simulink model "Hamiltonian_model"  (R2018b)
settings: Solver=FixedStepAuto  StartTime=0.0  StopTime=tsim  FixedStep=T  RelTol=1e-3
values from neighbouring files (symbols this model uses):
  a1 = 6.5035    [DoD_simulation.m]    (also in Hamiltonian_sim.m)
  a2 = 6.3853e-4    (= 0.00063853)    [DoD_simulation.m]    (also in Hamiltonian_sim.m)
  a3 = 0.0011    [DoD_simulation.m]    (also in Hamiltonian_sim.m)
  a4 = 0.0250    (= 0.025)    [DoD_simulation.m]    (also in Hamiltonian_sim.m)
  a5 = 0.1042    [DoD_simulation.m]    (also in Hamiltonian_sim.m)
  a6 = 0.0012    [DoD_simulation.m]    (also in Hamiltonian_sim.m)
  Aineq = [eye(N_MPC);-eye(N_MPC)]    [Hamiltonian_sim.m]
  B1 = 3.0021e3    (= 3002.1)    [DoD_simulation.m]    (also in Hamiltonian_sim.m)
  B2 = 986.7121    [DoD_simulation.m]    (also in Hamiltonian_sim.m)
  B3 = 210000    [DoD_simulation.m]    (also in Hamiltonian_sim.m)
  B4 = 19998    [DoD_simulation.m]    (also in Hamiltonian_sim.m)
  B5 = 35000    [DoD_simulation.m]    (also in Hamiltonian_sim.m)
  B6 = 19998    [DoD_simulation.m]    (also in Hamiltonian_sim.m)
  bineq = [fracU_max; -fracU_min]    [Hamiltonian_sim.m]
  Cm = [0, 0, 1, 0 ... (first row only)    [DoD_simulation.m]    (also in Hamiltonian_sim.m = [1, 0, 0, 0)
  Dm = [0;0;0]    [DoD_simulation.m]    (also in Hamiltonian_sim.m = [0; 0; 0])
  g = 9.82    [DoD_simulation.m]    (also in Hamiltonian_sim.m)
  Gamma = WW.'*[(BB.'*QQ + SS.')*(AA + BB*EE) + (BB.'*SS + RR)*EE, -(BB.'*QQ + SS.')*kron(ones(N_MPC+1,1),NN)]    [Hamiltonian_sim.m]
  Jo = 0.5*mo*(ro^2)    (= 0.000244290244743)    [DoD_simulation.m]    (also in Hamiltonian_sim.m)
  k = place(Ac,Bc,[p1 p2 p3])    [Hamiltonian_sim.m]
  Kc = zeros(1,length(idx))    [DoD_simulation.m]    (also in Hamiltonian_sim.m)
  Kw = 0.0086    [DoD_simulation.m]    (also in Hamiltonian_sim.m)
  Linv = L_H\eye(size(H,1))    [Hamiltonian_sim.m]
  Lo = dlqr(Aod.',Cm.',Qo,Ro).'    [DoD_simulation.m]
  mo = pi*(ro^2)*thick*p    (= 0.135716802635)    [DoD_simulation.m]    (also in Hamiltonian_sim.m)
  mup_init = [0; 0; theta0; phi0]    [DoD_simulation.m]    (also in Hamiltonian_sim.m)
  N = 98.78    [DoD_simulation.m]    (also in Hamiltonian_sim.m)
  n_in = size(Bcd,2)    [Hamiltonian_sim.m]
  n_out = size(Cc,1)    [Hamiltonian_sim.m]
  Nu = NN(end)    [DoD_simulation.m]    (also in Hamiltonian_sim.m)
  Nx = zeros(length(Cr),1)    [DoD_simulation.m]    (also in Hamiltonian_sim.m)
  opt = mpcqpsolverOptions    [Hamiltonian_sim.m]
  p1 = 0.7427    [DoD_simulation.m]    (also in Hamiltonian_sim.m = -4 + 0.5i)
  p2 = -0.2106    [DoD_simulation.m]    (also in Hamiltonian_sim.m = -4 - 0.5i)
  p3 = 1.121    [DoD_simulation.m]    (also in Hamiltonian_sim.m = -1.9)
  phi0 = 7.9*(pi/180)    (= 0.137881010908)    [DoD_simulation.m]    (also in Hamiltonian_sim.m = 0.0174532925199)
  Pp_init = 1e2*eye(4)    [DoD_simulation.m]    (also in Hamiltonian_sim.m = diag([1e0, 1e0, 1e0, 1e0]))
  Qo = diag([1e4, 1e2, 1e2, 1e-0])    [DoD_simulation.m]    (also in Hamiltonian_sim.m = diag([1e-10, 1e-10, 1e-10, 1e-10]))
  Ra = 2.5625    [DoD_simulation.m]    (also in Hamiltonian_sim.m)
  rh = 0.12    [DoD_simulation.m]    (also in Hamiltonian_sim.m)
  Ro = diag([1e-4, 1e-4, 9.0851e-04])    [DoD_simulation.m]    (also in Hamiltonian_sim.m = diag([1e3, 1e3, 1e3]))
  ro = 0.06    [DoD_simulation.m]    (also in Hamiltonian_sim.m)
  T = 0.01    [DoD_simulation.m]    (also in Hamiltonian_sim.m = 0.12)
  theta0 = 0*(pi/180)    (= 0)    [DoD_simulation.m]    (also in Hamiltonian_sim.m)
undefined symbols (not defined in the file or in its folder): Acd, Aod, Bcd, Bod, DiscIntNeverNeededParam
settings Model: Creator=timot  LastModifiedBy=timot
settings DebuggingCC: AlgebraicLoopMsg=none  LibraryContextMissingDiagnostic=none
settings SFSimCC: SimUseLocalCustomCode=off
settings RTWCC: RTWUseLocalCustomCode=off

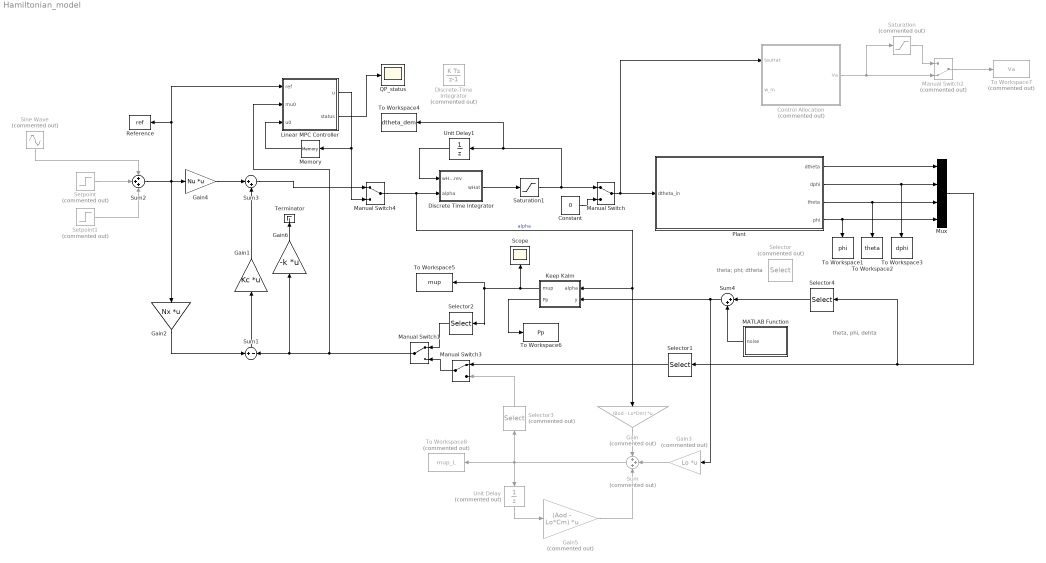
== system Hamiltonian_model ==
  note: theta; phi; dtheta
  note: theta, phi, dehta
  Constant : Constant  Value=0
  Control Allocation : MATLAB Function  Commented=on  TreatAsAtomicUnit=on
  Discrete Time Integrator : MATLAB Function  TreatAsAtomicUnit=on
  Discrete-Time Integrator : DiscreteIntegrator  Commented=on  SampleTime=-1  ICPrevOutput=DiscIntNeverNeededParam  ICPrevScaledInput=DiscIntNeverNeededParam
  Gain : Gain  Commented=on  Gain=(Bod - Lo*Dm)  Multiplication=Matrix(K*u)
  Gain1 : Gain  Gain=Kc  Multiplication=Matrix(K*u)
  Gain2 : Gain  Gain=Nx  Multiplication=Matrix(K*u)
  Gain3 : Gain  Commented=on  Gain=Lo  Multiplication=Matrix(K*u)
  Gain4 : Gain  Gain=Nu  Multiplication=Matrix(K*u)
  Gain5 : Gain  Commented=on  Gain=(Aod - Lo*Cm)  Multiplication=Matrix(K*u)
  Gain6 : Gain  Gain=-k  Multiplication=Matrix(K*u)
  Keep Kalm : Subsystem
  Linear MPC Controller : MATLAB Function  TreatAsAtomicUnit=on  SystemSampleTime=T
  MATLAB Function : MATLAB Function  TreatAsAtomicUnit=on
  Manual Switch{,1,3..4} (4 alike) : ManualSwitch
  Manual Switch2 : ManualSwitch  Commented=on  CurrentSetting=0
  Memory : Memory  InitialCondition=zeros(n_out,1)  InheritSampleTime=on
  Mux : Mux
  Plant : Subsystem
  QP_status : Scope
  Reference : ToWorkspace  VariableName=ref  SaveFormat=Structure With Time  SampleTime=-1
  Saturation : Saturate  Commented=on  UpperLimit=6  LowerLimit=-6
  Saturation1 : Saturate  UpperLimit=10  LowerLimit=-10
  Scope : Scope
  Selector : Selector  Commented=on  InputPortWidth=4  IndexOptions=Index vector (dialog)  Indices=[3, 4, 1]  OutputSizes=1
  Selector1 : Selector  InputPortWidth=4  IndexOptions=Index vector (dialog)  Indices=[1 2 4]  OutputSizes=1
  Selector2 : Selector  InputPortWidth=4  IndexOptions=Index vector (dialog)  Indices=[1 2 4]  OutputSizes=1
  Selector3 : Selector  Commented=on  InputPortWidth=4  IndexOptions=Index vector (dialog)  Indices=[1 2 4]  OutputSizes=1
  Selector4 : Selector  InputPortWidth=4  IndexOptions=Index vector (dialog)  Indices=[1 3 4]  OutputSizes=1
  Setpoint : Step  Commented=on  Time=3  After=2*pi  SampleTime=0
  Setpoint1 : Step  Commented=on  Time=6  After=-pi  SampleTime=0
  Sine Wave : Sin  Commented=on  Amplitude=3  SampleTime=0
  Sum : Sum  Commented=on  Inputs=+++
  Sum1 : Sum  Inputs=+|-
  Sum2 : Sum  Inputs=+++
  Sum3 : Sum  Inputs=|++
  Sum4 : Sum  Inputs=|++
  Terminator : Terminator
  To Workspace1 : ToWorkspace  VariableName=phi  SaveFormat=Structure With Time  SampleTime=-1
  To Workspace2 : ToWorkspace  VariableName=theta  SaveFormat=Structure With Time  SampleTime=-1
  To Workspace3 : ToWorkspace  VariableName=dphi  SaveFormat=Structure With Time  SampleTime=-1
  To Workspace4 : ToWorkspace  VariableName=dtheta_dem  SaveFormat=Structure With Time  SampleTime=-1
  To Workspace5 : ToWorkspace  VariableName=mup  SaveFormat=Structure With Time  SampleTime=-1
  To Workspace6 : ToWorkspace  VariableName=Pp  SaveFormat=Structure With Time  SampleTime=-1
  To Workspace7 : ToWorkspace  Commented=on  VariableName=Va  SaveFormat=Structure With Time  SampleTime=-1
  To Workspace8 : ToWorkspace  Commented=on  VariableName=mup_L  SaveFormat=Structure With Time  SampleTime=-1
  Unit Delay : UnitDelay  Commented=on  InitialCondition=mup_init  SampleTime=T
  Unit Delay1 : UnitDelay  SampleTime=-1
  wires:
  Gain4/1 -> Sum3/1
  Sum2/1 -> Gain4/1, Gain2/1, Linear MPC Controller/1(ref), Reference/1
  Sum1/1 -> Gain1/1
  Gain2/1 -> Sum1/1
  Gain1/1 -> Sum3/2
  Constant/1 -> Manual Switch/2
  Keep Kalm/1(mup) -> To Workspace5/1, Selector2/1, Scope/1
  Keep Kalm/2(Pp) -> To Workspace6/1
  Control Allocation/1(Va) -> Manual Switch2/2, Saturation/1
  Setpoint/1 -> Sum2/2
  Setpoint1/1 -> Sum2/3
  Sine Wave/1 -> Sum2/1
  Manual Switch2/1 -> To Workspace7/1
  Saturation/1 -> Manual Switch2/1
  Manual Switch3/1 -> Manual Switch1/2
  Gain/1 -> Sum/1
  Gain5/1 -> Sum/3
  Gain3/1 -> Sum/2
  Unit Delay/1 -> Gain5/1
  Mux/1 -> Selector4/1, Selector1/1
  MATLAB Function/1(noise) -> Sum4/2
  Sum4/1 -> Gain3/1, Keep Kalm/2(y)
  Plant/1("dtheta ") -> Mux/1
  Plant/2(dphi) -> To Workspace3/1, Mux/2
  Plant/3(theta) -> To Workspace2/1, Mux/3
  Plant/4(phi) -> To Workspace1/1, Mux/4
  Manual Switch/1 -> Control Allocation/1(tauHat), Plant/1(dtheta_in)
  Selector1/1 -> Manual Switch3/1
  Discrete Time Integrator/1(wHat) -> Saturation1/1
  Selector2/1 -> Manual Switch1/1
  Sum/1 -> To Workspace8/1, Selector3/1, Unit Delay/1
  Selector3/1 -> Manual Switch3/2
  Unit Delay1/1 -> Discrete Time Integrator/1(wHat_prev)
  Selector4/1 -> Sum4/1
  Sum3/1 -> Manual Switch4/1
  Manual Switch4/1 -> Keep Kalm/1(alpha), Gain/1, Discrete Time Integrator/2(alpha)  "alpha"
  Manual Switch1/1 -> Linear MPC Controller/2(mu0), Gain6/1, Sum1/2
  Memory/1 -> Linear MPC Controller/3(u0)
  Linear MPC Controller/1(u) -> Memory/1, Manual Switch4/2
  Linear MPC Controller/2(status) -> QP_status/1
  Gain6/1 -> Terminator/1
  Saturation1/1 -> To Workspace4/1, Unit Delay1/1, Manual Switch/1

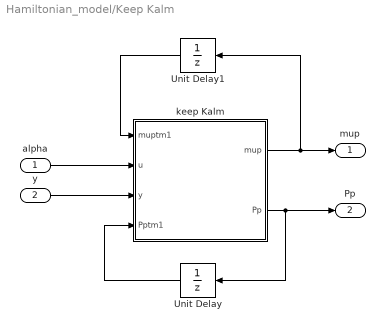
== system Hamiltonian_model/Keep Kalm ==
  alpha : Inport
  y : Inport  Port=2
  Unit Delay : UnitDelay  InitialCondition=Pp_init  SampleTime=-1
  Unit Delay1 : UnitDelay  InitialCondition=mup_init  SampleTime=-1
  keep Kalm : MATLAB Function  TreatAsAtomicUnit=on
  mup : Outport
  Pp : Outport  Port=2
  wires:
  keep Kalm/2(Pp) -> Unit Delay/1, Pp/1
  alpha/1 -> keep Kalm/2(u)
  keep Kalm/1(mup) -> mup/1, Unit Delay1/1
  Unit Delay/1 -> keep Kalm/4(Pptm1)
  Unit Delay1/1 -> keep Kalm/1(muptm1)
  y/1 -> keep Kalm/3(y)

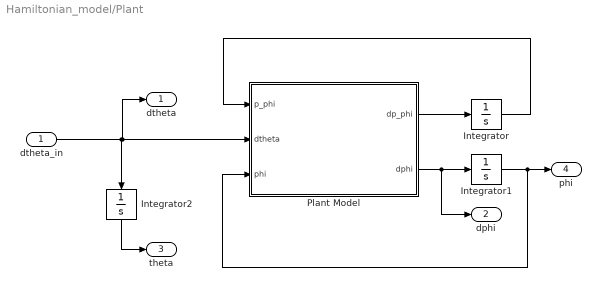
== system Hamiltonian_model/Plant ==
  dtheta_in : Inport
  Integrator : Integrator
  Integrator1 : Integrator  InitialCondition=phi0
  Integrator2 : Integrator  InitialCondition=theta0
  "Plant Model " : MATLAB Function  TreatAsAtomicUnit=on
  "dtheta " : Outport
  dphi : Outport  Port=2
  theta : Outport  Port=3
  phi : Outport  Port=4
  wires:
  "Plant Model "/1(dp_phi) -> Integrator/1
  Integrator/1 -> "Plant Model "/1(p_phi)
  dtheta_in/1 -> "dtheta "/1, "Plant Model "/2(dtheta), Integrator2/1
  Integrator2/1 -> theta/1
  "Plant Model "/2(dphi) -> dphi/1, Integrator1/1
  Integrator1/1 -> "Plant Model "/3(phi), phi/1

== matlab function Hamiltonian_model/Keep Kalm/keep Kalm ==
  data: muptm1 input; u input; y input; Pptm1 input; Cm parameter; Bod parameter; Qo parameter; Ro parameter; Aod parameter; Dm parameter; mup output; Pp output
function [mup, Pp] = fcn(muptm1, u, y, Pptm1, Cm, Bod, Qo, Ro, Aod, Dm)
% % Update with new measurement
% muf = muptm1 + Pptm1*Cm'*((Cm*Pptm1*Cm' + Ro)\(y - Cm*muptm1 - Dm*u));
% Pf = Pptm1 - Pptm1*Cm'*((Cm*Pptm1*Cm' + Ro)\(Cm*Pptm1));
% 
% % Predict Forward
% mup = Aod*muf + Bod*u;
% Pp = Aod*Pf*Aod' + Qo;

n = length(Aod);

% Optimal Kalman Gain
Kk = Pptm1*Cm.'/(Cm*Pptm1*Cm.' + Ro);

% Correct prediction using measurement
muf = muptm1 + Kk*(y - Cm*muptm1 - Dm*u);
% muf = muptm1 + Kk*(y - Cm*muptm1);

% Compute new covariance
Pf = (eye(n) - Kk*Cm)*Pptm1*(eye(n) - Kk*Cm).' + Kk*Ro*Kk.';

% Predict forward
% mup = Aod*muf;
mup = Aod*muf + Bod*u;

% Update prediction covariance
Pp = Aod*Pf*Aod.' + Qo;




% muf = mup(:,t) + Pp(:,:,t)*C'*((C*Pp(:,:,t)*C' + R)\(mup(:,t) - C*mup(:,t) - D*u(:,t)));
% Pf(:,:,t) = Pp(:,:,t) - Pp(:,:,t)*C'*((C*Pp(:,:,t)*C' + R)\(C*Pp(:,:,t)));
% %Predict forward
% mup(:,t+1) = A*muf(:,t) + B*u(:,t);
% Pp(:,:,t+1) = A*Pf(:,:,t)*A' + Q;
% 
%

== matlab function Hamiltonian_model/Plant/Plant Model  ==
  data: p_phi input; dtheta input; dp_phi output; dphi output; phi input; mo parameter; g parameter; rh parameter; ro parameter; Jo parameter
function [dp_phi, dphi] = fcn(p_phi, dtheta, phi, mo, g, rh, ro, Jo)

dp_phi = mo*g*(rh+ro)*sin(phi);

dphi = (p_phi + Jo*((rh^2)/(ro^2))*dtheta)/(mo*((rh+ro)^2) + Jo*((rh^2)/(ro^2)));

== matlab function Hamiltonian_model/Control Allocation ==
  data: tauHat input; Va output; w_m input; Ra parameter; Kw parameter; N parameter; a1 parameter; a2 parameter; a3 parameter; B1 parameter; B2 parameter; B3 parameter; a4 parameter; a5 parameter; a6 parameter; B4 parameter; B5 parameter; B6 parameter; p1 parameter; p2 parameter; p3 parameter
function Va = controlAllocation(tauHat, w_m, Ra, Kw, N, a1, a2, a3, B1, B2,...
    B3, a4, a5, a6, B4, B5, B6, p1, p2, p3)
% Correct velocity
w_m = w_m.*N;

% Heaviside functions
heavi_p =@(x) 1./(1 + exp(-2.*50.*x));
heavi_m =@(x) 1./(1 + exp(-2.*50.*-x));

% Friction function
tauF = (a1.*(tanh(B1.*w_m) - tanh(B2.*w_m)) + a2.*tanh(B3.*w_m) + a3.*w_m).*heavi_p(w_m)...
                + (a4.*(tanh(B4.*w_m) - tanh(B5.*w_m)) + a5.*tanh(B6.*w_m) + a6.*w_m).*heavi_m(w_m);

% Motor torque
Tm = tauHat - tauF;

% Current
Ia =  p1.*Tm.^3 + p2.*Tm.^2 + p3.*Tm;

% Voltage
Va = Kw.*w_m + Ra.*Ia;

== matlab function Hamiltonian_model/MATLAB Function ==
  data: noise output
function noise = noisyboi()
noise = 0.00000001.*randn(3,1);

== matlab function Hamiltonian_model/Discrete Time Integrator ==
  data: wHat_prev input; wHat output; alpha input; T parameter
function wHat = fcn(wHat_prev, alpha, T)
wHat = wHat_prev + T*alpha;

== matlab function Hamiltonian_model/Linear MPC Controller ==
  settings: updateMethod=DISCRETE  sampleTime=T
  data: ref input; u output size=1; mu0 input; Linv parameter; opt parameter; n_in parameter size=1; u0 input; status output; Gamma parameter; Acd parameter; Bcd parameter; Aineq parameter; bineq parameter
function [u, status] = MPC(ref, mu0, Linv, opt, n_in, u0, Gamma, Acd, Bcd, Aineq, bineq)
%#codegen

% Predict state at next time step
mu1 = Acd*mu0 + Bcd*u0;

% Compute linear coefficient of QP
kk = [mu1; u0; ref];
g = Gamma*kk;

iA0 = false(size(Aineq,1),1);   % Initial active constraints

% The KWIK algorithm defines inequality constraints as Ax >= b rather than 
% Ax <= b, as in the quadprog command.
[uMPC, status] = mpcqpsolver(Linv, g, -Aineq, -bineq, [], zeros(0,1), iA0, opt);

% Return next control action
u = uMPC(1:n_in);
